simulink model "ProjectDamp"  (R2018b)
settings: Solver=VariableStepAuto  StartTime=0.0  StopTime=10.0  RelTol=1e-3
values from neighbouring files (symbols this model uses):
  b = 5    [runDamp.m]
  F = 1    [runDamp.m]
  k = 20    [runDamp.m]
  M = 1    [runDamp.m]
settings Model: Creator=Ismael  LastModifiedBy=Ismael

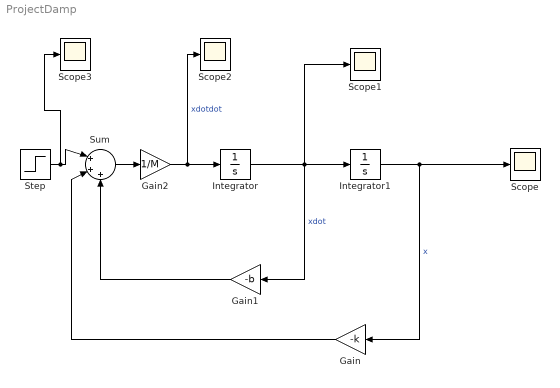
== system ProjectDamp ==
  Gain : Gain  Gain=-k
  Gain1 : Gain  Gain=-b
  Gain2 : Gain  Gain=1/M
  Integrator : Integrator
  Integrator1 : Integrator
  Scope{,1..3} (4 alike) : Scope
  Step : Step  After=F  SampleTime=0
  Sum : Sum  Inputs=|+++
  wires:
  Integrator/1 -> Scope1/1, Gain1/1, Integrator1/1  "xdot"
  Integrator1/1 -> Scope/1, Gain/1  "x"
  Gain1/1 -> Sum/3
  Gain/1 -> Sum/2
  Step/1 -> Scope3/1, Sum/1
  Sum/1 -> Gain2/1
  Gain2/1 -> Scope2/1, Integrator/1  "xdotdot"
